simulink model "mavlink_task"  (Simulink 3.00)
undefined symbols (not defined in the file): Double, F64, I32, Long
libraries: mathlib x22, MAVLink_library x7, genlib x4, mavlinklib x3, logiclib x3, matrixlib x2, analoglib x2, speclib x1, arclib x1
settings Model: MaskType=REX sequence  MaskIconFrame=on  MaskIconOpaque=on  MaskIconRotate=none  MaskIconUnits=autoscale

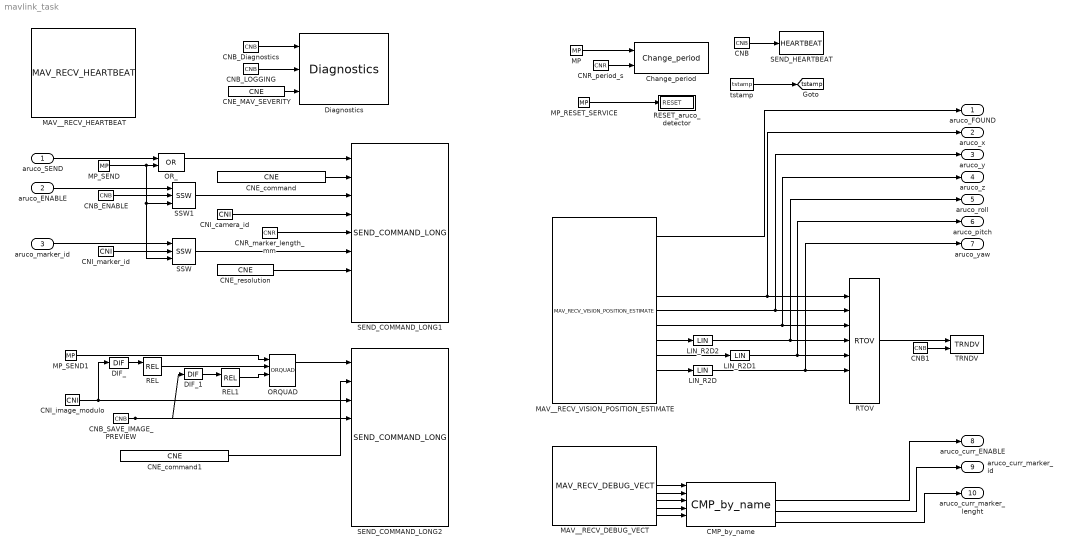
== system mavlink_task ==
  aruco_SEND : Inport  Port=1  OutDataTypeStr=Inherit: auto
  aruco_ENABLE : Inport  Port=2  OutDataTypeStr=Inherit: auto
  aruco_marker_id : Inport  Port=3  OutDataTypeStr=Inherit: auto
  CMP_by_name : MAVLink_library/CMP_by_name  name=aruco
  CNB : mathlib/CNB  YCN=on
  CNB1 : mathlib/CNB  YCN=off
  CNB_Diagnostics : mathlib/CNB  YCN=off
  CNB_ENABLE : mathlib/CNB  YCN=on
  CNB_LOGGING : mathlib/CNB  YCN=off
  CNB_SAVE_IMAGE_PREVIEW : mathlib/CNB  YCN=off
  CNE_MAV_SEVERITY : mathlib/CNE  yenum=6: Info  pupstr=3: Error|4: Warning|6: Info|7: Verbose
  CNE_command : mathlib/CNE  yenum=31010: MAV_CMD_USER_1  pupstr=31010: MAV_CMD_USER_1|31011: MAV_CMD_USER_2|31012: MAV_CMD_USER_3|31013: MAV_CMD_USER_4
  CNE_command1 : mathlib/CNE  yenum=31012: MAV_CMD_USER_3  pupstr=31010: MAV_CMD_USER_1|31011: MAV_CMD_USER_2|31012: MAV_CMD_USER_3|31013: MAV_CMD_USER_4
  CNE_resolution : mathlib/CNE  yenum=4: 1920x1080  pupstr=0: 640x480|1: 800x600|2: 1280x720|3: 1280x960|4: 1920x1080|5: 1920x1200
  CNI_camera_id : mathlib/CNI  icn=0  vtype=4: Long (I32)
  CNI_image_modulo : mathlib/CNI  icn=0  vtype=4: Long (I32)
  CNI_marker_id : mathlib/CNI  icn=12  vtype=4: Long (I32)
  CNR_marker_length_mm : mathlib/CNR  ycn=20
  CNR_period_s : mathlib/CNR  ycn=5
  Change_period : MAVLink_library/Change_period  TgtSysID=254  TgtCompID=173
  DIF_ : mathlib/DIF  ISSF=off
  DIF_1 : mathlib/DIF  ISSF=off
  Diagnostics : MAVLink_library/Diagnostics  SrcSystemID=254  SrcComponentID=173
  LIN_R2D : mathlib/LIN  u1=0  y1=0  u2=3.14159265359  y2=180
  LIN_R2D1 : mathlib/LIN  u1=0  y1=0  u2=3.14159265359  y2=180
  LIN_R2D2 : mathlib/LIN  u1=0  y1=0  u2=3.14159265359  y2=180
  MAV__RECV_DEBUG_VECT : mavlinklib/MAV_RECV_DEBUG_VECT  SrcSystemID=254  SrcComponentID=173  TgtSystemID=-1  TgtComponentID=-1  TimeoutMS=1000
  MAV__RECV_HEARTBEAT : mavlinklib/MAV_RECV_HEARTBEAT  SrcSystemID=254  SrcComponentID=173  TgtSystemID=-1  TgtComponentID=-1  TimeoutMS=0
  MAV__RECV_VISION_POSITION_ESTIMATE : mavlinklib/MAV_RECV_VISION_POSITION_ESTIMATE  SrcSystemID=254  SrcComponentID=173  TgtSystemID=-1  TgtComponentID=-1  TimeoutMS=1000
  MP : genlib/MP  BSTATE=off  pwidth=1  RPTF=off
  MP_RESET_SERVICE : genlib/MP  BSTATE=off  pwidth=1  RPTF=off
  MP_SEND : genlib/MP  BSTATE=off  pwidth=1  RPTF=off
  MP_SEND1 : genlib/MP  BSTATE=off  pwidth=1  RPTF=off
  ORQUAD : logiclib/ORQUAD  nl=0
  OR_ : logiclib/OR
  REL : mathlib/REL  irel=2: inequality (!=)
  REL1 : mathlib/REL  irel=2: inequality (!=)
  RESET_aruco_detector : Subsystem
      mask Type: REX sequence
  RTOV : matrixlib/RTOV  nmax=8  offset=0  n=8  etype=8: Double (F64)
  SEND_COMMAND_LONG1 : MAVLink_library/SEND_COMMAND_LONG  TgtSysID=254  TgtCompID=173  Timeout=1
  SEND_COMMAND_LONG2 : MAVLink_library/SEND_COMMAND_LONG  TgtSysID=254  TgtCompID=173  Timeout=1
  SEND_HEARTBEAT : MAVLink_library/HEARTBEAT
      mask Type: REX sequence
  SSW : analoglib/SSW
  SSW1 : analoglib/SSW
  TRNDV : arclib/TRNDV  n=6  l=1000  btype=8: Double (F64)  pfac=1  afac=0  arc=0  id=1  Title=Trend Title  timesrc=1: CORETIMER  ViewConfig="{\"View\":{\"Data\":{\"History\":13.107200000000004,\"XAxisTimeFormat\":66},\"PropertiesModel\":[{\"Id\":0,\"Items\":[{\"Color\":\"#ff0000\",\"Id\":0,\"IsActive\":true,\"LineWidth\":2,\"Name\":\"X\",\"SceneNumber\":2},{\"Color\":\"#669900\",\"Id\":1,\"IsActive\":true,\"LineWidth\":2,\"Name\":\"Y\",\"SceneNumber\":2},{\"Color\":\"#000099\",\"Id\":2,\"IsActive\":true,\"LineWidth\":2,\"Name\":\"Z\",\"SceneNumber\":2},{\"Color\":\"#9966cc\",\"Id\":3,\"IsActive\":true,\"LineWidth\":2,\"Name\":\"roll\",\"SceneNumber\":2},{\"Color\":\"#339999\",\"Id\":4,\"IsActive\":true,\"LineWidth\":2,\"Name\":\"pitch\",\"SceneNumber\":2},{\"Color\":\"#996600\",\"Id\":5,\"IsActive\":true,\"LineWidth\":2,\"Name\":\"yaw\",\"SceneNumber\":2}]}],\"Scenes\":[{\"Id\":2}],\"sync\":false}}"
  tstamp : MAVLink_library/tstamp
      mask Type: REX sequence
  aruco_FOUND : Outport  Port=1  OutDataTypeStr=Inherit: auto
  aruco_x : Outport  Port=2  OutDataTypeStr=Inherit: auto
  aruco_y : Outport  Port=3  OutDataTypeStr=Inherit: auto
  aruco_z : Outport  Port=4  OutDataTypeStr=Inherit: auto
  aruco_roll : Outport  Port=5  OutDataTypeStr=Inherit: auto
  aruco_pitch : Outport  Port=6  OutDataTypeStr=Inherit: auto
  aruco_yaw : Outport  Port=7  OutDataTypeStr=Inherit: auto
  aruco_curr_ENABLE : Outport  Port=8  OutDataTypeStr=Inherit: auto
  aruco_curr_marker_id : Outport  Port=9  OutDataTypeStr=Inherit: auto
  aruco_curr_marker_lenght : Outport  Port=10  OutDataTypeStr=Inherit: auto
  tag scope: tstamp=global
  wires:
  CMP_by_name/2 -> aruco_curr_ENABLE/1
  CMP_by_name/3 -> aruco_curr_marker_id/1
  CMP_by_name/4 -> aruco_curr_marker_lenght/1
  CNB/1 -> SEND_HEARTBEAT/1
  CNB1/1 -> TRNDV/2
  CNB_Diagnostics/1 -> Diagnostics/1
  CNB_ENABLE/1 -> SSW1/2
  CNB_LOGGING/1 -> Diagnostics/2
  CNB_SAVE_IMAGE_PREVIEW/1 -> DIF_1/1, SEND_COMMAND_LONG2/4
  CNE_MAV_SEVERITY/1 -> Diagnostics/3
  CNE_command/1 -> SEND_COMMAND_LONG1/2
  CNE_command1/1 -> SEND_COMMAND_LONG2/2
  CNE_resolution/1 -> SEND_COMMAND_LONG1/7
  CNI_camera_id/1 -> SEND_COMMAND_LONG1/4
  CNI_image_modulo/1 -> DIF_/1, SEND_COMMAND_LONG2/3
  CNI_marker_id/1 -> SSW/2
  CNR_marker_length_mm/1 -> SEND_COMMAND_LONG1/5
  CNR_period_s/1 -> Change_period/2
  DIF_/1 -> REL/1
  DIF_1/1 -> REL1/1
  LIN_R2D/1 -> RTOV/7, aruco_yaw/1
  LIN_R2D1/1 -> RTOV/6, aruco_pitch/1
  LIN_R2D2/1 -> RTOV/5, aruco_roll/1
  MAV__RECV_DEBUG_VECT/5 -> CMP_by_name/1
  MAV__RECV_DEBUG_VECT/6 -> CMP_by_name/2
  MAV__RECV_DEBUG_VECT/7 -> CMP_by_name/3
  MAV__RECV_DEBUG_VECT/8 -> CMP_by_name/4
  MAV__RECV_DEBUG_VECT/9 -> CMP_by_name/5
  MAV__RECV_VISION_POSITION_ESTIMATE/2 -> aruco_FOUND/1
  MAV__RECV_VISION_POSITION_ESTIMATE/6 -> RTOV/2, aruco_x/1
  MAV__RECV_VISION_POSITION_ESTIMATE/7 -> RTOV/3, aruco_y/1
  MAV__RECV_VISION_POSITION_ESTIMATE/8 -> RTOV/4, aruco_z/1
  MAV__RECV_VISION_POSITION_ESTIMATE/9 -> LIN_R2D2/1
  MAV__RECV_VISION_POSITION_ESTIMATE/10 -> LIN_R2D1/1
  MAV__RECV_VISION_POSITION_ESTIMATE/11 -> LIN_R2D/1
  MP/1 -> Change_period/1
  MP_RESET_SERVICE/1 -> RESET_aruco_detector/1(RESET)
  MP_SEND/1 -> OR_/2, SSW/3, SSW1/3
  MP_SEND1/1 -> ORQUAD/1
  ORQUAD/1 -> SEND_COMMAND_LONG2/1
  OR_/1 -> SEND_COMMAND_LONG1/1
  REL/1 -> ORQUAD/2
  REL1/1 -> ORQUAD/3
  RTOV/1 -> TRNDV/1
  SSW/1 -> SEND_COMMAND_LONG1/6
  SSW1/1 -> SEND_COMMAND_LONG1/3
  aruco_ENABLE/1 -> SSW1/1
  aruco_SEND/1 -> OR_/1
  aruco_marker_id/1 -> SSW/1
  tstamp/1 -> [tstamp]

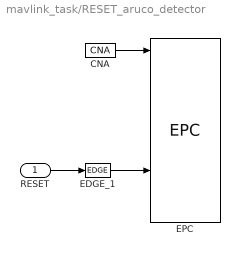
== system mavlink_task/RESET_aruco_detector ==
  RESET : Inport  Port=1  OutDataTypeStr=Inherit: auto
  CNA : matrixlib/CNA  TRN=off  nmax=100  etype=8: Double (F64)  acn=[0 1 2 3]
  EDGE_1 : logiclib/EDGE  iedge=1: Rising edge
  EPC : speclib/EPC  cmd=systemctl restart aruco-detector.service  ifns=epc_uVec1  ofns=epc_yVec1  sl=85  ifm=1  format=1: Space-delimited values  nmax=100
  wires:
  CNA/1 -> EPC/1
  EDGE_1/1 -> EPC/9
  RESET/1 -> EDGE_1/1
